simulink model "sim_podlogowa_model_tkz"  (R2021b)
settings: Solver=VariableStepAuto  StartTime=0.0  StopTime=10.0  MaxStep=5  RelTol=1e-3
undefined symbols (not defined in the file): czas_skoku_10pro, dspr, k, T0_klasyczna, T_klasyczna
settings Model: Creator=adams  LastModifiedBy=adams

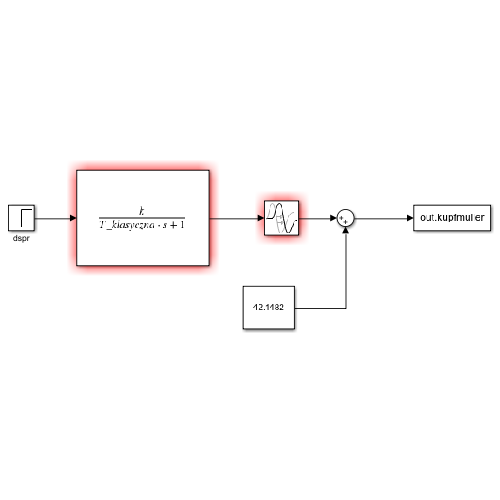
[thumbnail: Simulink's stored preview of the top-level diagram]
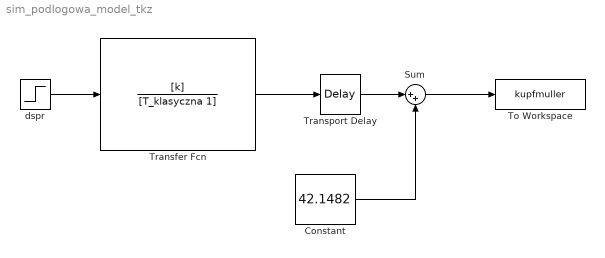
== system sim_podlogowa_model_tkz ==
  Constant : Constant  Value=42.1482
  Sum : Sum  Inputs=|++
  To Workspace : ToWorkspace  VariableName=kupfmuller  SampleTime=-1
  Transfer Fcn : TransferFcn  Numerator=[k]  Denominator=[T_klasyczna 1]
  Transport Delay : TransportDelay  DelayTime=T0_klasyczna  BufferSize=32768
  dspr : Step  Time=czas_skoku_10pro  After=dspr  SampleTime=0
  wires:
  Sum/1 -> To Workspace/1
  Constant/1 -> Sum/2
  Transport Delay/1 -> Sum/1
  Transfer Fcn/1 -> Transport Delay/1
  dspr/1 -> Transfer Fcn/1
